simulink model "mcb_pmsm_param_est_f28379d"  (R2024b)
settings: Solver=FixedStepDiscrete  StartTime=0.0  StopTime=12  RelTol=1e-3  EnableMultiTasking=on
InitFcn:
  | mcb_pmsm_param_est_f28379d_data;
values from neighbouring files (symbols this model uses):
  dataType = 'single'    [mcb_pmsm_param_est_f28379d_data.m]
  inverter = evalin('base','inverter')    [mcb_param_est_StopFunc.m]    (also in mcb_pmsm_param_est_f28379d_data.m = mcb_updateInverterParameters(motor,inverter,target))
  target = mcb_SetProcessorDetails('F28379D',PWM_frequency)    [mcb_pmsm_param_est_f28379d_data.m]
  Ts = T_pwm    (= 5e-05)    [mcb_pmsm_param_est_f28379d_data.m]
  Ts_motor = T_pwm/2    (= 2.5e-05)    [mcb_pmsm_param_est_f28379d_data.m]
undefined symbols (not defined in the file or in its folder): Down, GPTRIP1SEL, GPTRIP2SEL, motor, TZ1, TZ2, Up
libraries: simulink x14, c2802xlib x8, c280xlib x5, mcbpmsmparamestlib x5, c2837xDlib x4, mcbpositiondecoderlib x3, svdschedulerlib x2, autolibpmsminterior x2, mcbplantlib x1, mcbcontrolslib x1, svdutilitieslib x1
(part 3 of 3)

== system mcb_pmsm_param_est_f28379d/Serial Receive/Variant Subsystem/Codegen/Subsystem/Switch Case Action Subsystem3 ==
  In1 : Inport
  Action Port : ActionPort
  Out1 : Outport
  wires:
  In1/1 -> Out1/1

== system mcb_pmsm_param_est_f28379d/Serial Receive/Variant Subsystem/Codegen/Subsystem/Switch Case Action Subsystem4 ==
  In1 : Inport
  Action Port : ActionPort
  Out1 : Outport
  wires:
  In1/1 -> Out1/1

== system mcb_pmsm_param_est_f28379d/Serial Receive/Variant Subsystem/Codegen/Subsystem/Switch Case Action Subsystem5 ==
  In1 : Inport
  Action Port : ActionPort
  Out1 : Outport
  wires:
  In1/1 -> Out1/1

== system mcb_pmsm_param_est_f28379d/Serial Receive/Variant Subsystem/Codegen/Subsystem/Switch Case Action Subsystem6 ==
  In1 : Inport
  Action Port : ActionPort
  Out1 : Outport
  wires:
  In1/1 -> Out1/1

== system mcb_pmsm_param_est_f28379d/Serial Receive/Variant Subsystem/Codegen/Subsystem/Switch Case Action Subsystem7 ==
  In1 : Inport
  Action Port : ActionPort
  Out1 : Outport
  wires:
  In1/1 -> Out1/1

== system mcb_pmsm_param_est_f28379d/Serial Receive/Variant Subsystem/Codegen/Subsystem/Switch Case Action Subsystem8 ==
  In1 : Inport
  Action Port : ActionPort  ActionPortLabel=case [ 21 ]:
  Out1 : Outport
  wires:
  In1/1 -> Out1/1

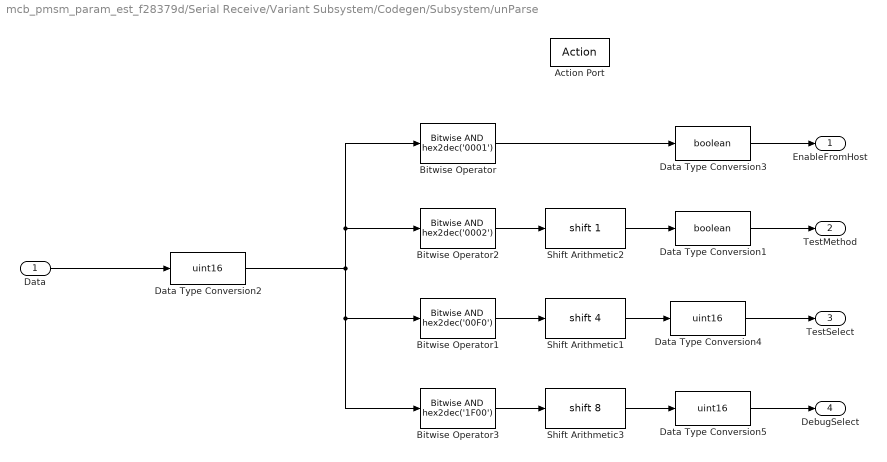
== system mcb_pmsm_param_est_f28379d/Serial Receive/Variant Subsystem/Codegen/Subsystem/unParse ==
  Data : Inport
  Action Port : ActionPort  ActionPortLabel=case [ 22 ]:
  Bitwise Operator : simulink/Logic and Bit Operations/Bitwise Operator  logicop=AND  UseBitMask=on  BitMask=hex2dec('0001')  BitMaskRealWorld=Stored Integer
  Bitwise Operator1 : simulink/Logic and Bit Operations/Bitwise Operator  logicop=AND  UseBitMask=on  BitMask=hex2dec('00F0')  BitMaskRealWorld=Stored Integer
  Bitwise Operator2 : simulink/Logic and Bit Operations/Bitwise Operator  logicop=AND  UseBitMask=on  BitMask=hex2dec('0002')  BitMaskRealWorld=Stored Integer
  Bitwise Operator3 : simulink/Logic and Bit Operations/Bitwise Operator  logicop=AND  UseBitMask=on  BitMask=hex2dec('1F00')  BitMaskRealWorld=Stored Integer
  Data Type Conversion1 : DataTypeConversion  OutDataTypeStr=boolean  RndMeth=Simplest  SaturateOnIntegerOverflow=off
  Data Type Conversion2 : DataTypeConversion  OutDataTypeStr=uint16  RndMeth=Simplest  SaturateOnIntegerOverflow=off
  Data Type Conversion3 : DataTypeConversion  OutDataTypeStr=boolean  RndMeth=Simplest  SaturateOnIntegerOverflow=off
  Data Type Conversion4 : DataTypeConversion  OutDataTypeStr=uint16  RndMeth=Simplest  SaturateOnIntegerOverflow=off
  Data Type Conversion5 : DataTypeConversion  OutDataTypeStr=uint16  RndMeth=Simplest  SaturateOnIntegerOverflow=off
  Shift Arithmetic1 : ArithShift  BitShiftNumber=4
  Shift Arithmetic2 : ArithShift  BitShiftNumber=1
  Shift Arithmetic3 : ArithShift  BitShiftNumber=8
  EnableFromHost : Outport
  TestMethod : Outport  Port=2
  TestSelect : Outport  Port=3
  DebugSelect : Outport  Port=4
  wires:
  Shift Arithmetic3/1 -> Data Type Conversion5/1
  Data Type Conversion5/1 -> DebugSelect/1
  Bitwise Operator3/1 -> Shift Arithmetic3/1
  Data Type Conversion2/1 -> Bitwise Operator1/1, Bitwise Operator3/1, Bitwise Operator/1, Bitwise Operator2/1
  Bitwise Operator1/1 -> Shift Arithmetic1/1
  Data/1 -> Data Type Conversion2/1
  Bitwise Operator/1 -> Data Type Conversion3/1
  Data Type Conversion4/1 -> TestSelect/1
  Shift Arithmetic1/1 -> Data Type Conversion4/1
  Data Type Conversion3/1 -> EnableFromHost/1
  Bitwise Operator2/1 -> Shift Arithmetic2/1
  Shift Arithmetic2/1 -> Data Type Conversion1/1
  Data Type Conversion1/1 -> TestMethod/1

== system mcb_pmsm_param_est_f28379d/Hardware Init/Variant Subsystem/Code Generation/Calculate ADC Offset /For Iterator Subsystem/If Action Subsystem ==
  In1 : Inport
  In2 : Inport  Port=2
  Action Port : ActionPort
  Memory : Memory  InheritSampleTime=on
  Memory1 : Memory  InheritSampleTime=on
  Sum : Sum
  Sum1 : Sum
  Out1 : Outport
  Out2 : Outport  Port=2
  wires:
  In1/1 -> Sum/1
  Sum/1 -> Out1/1, Memory/1
  In2/1 -> Sum1/1
  Memory/1 -> Sum/2
  Sum1/1 -> Out2/1, Memory1/1
  Memory1/1 -> Sum1/2

== system mcb_pmsm_param_est_f28379d/Parameter Estimation/Output HW Drivers/SCI Drivers/Codegen/Data_Conditioning_Tx/Data_Type_Fixed_Point ==
  In1 : Inport
  Data Type Conversion : DataTypeConversion  OutDataTypeStr=fixdt(1,32,28)  RndMeth=Simplest  SaturateOnIntegerOverflow=off
  Data Type Conversion3 : DataTypeConversion  OutDataTypeStr=uint32  ConvertRealWorld=Stored Integer (SI)  RndMeth=Simplest  SaturateOnIntegerOverflow=off
  Data_Log : Outport
  wires:
  In1/1 -> Data Type Conversion/1
  Data Type Conversion3/1 -> Data_Log/1
  Data Type Conversion/1 -> Data Type Conversion3/1

== system mcb_pmsm_param_est_f28379d/Parameter Estimation/Output HW Drivers/SCI Drivers/Codegen/Data_Conditioning_Tx/Data_Type_Float ==
  In1 : Inport
  Byte Pack : svdutilitieslib/Byte Pack  maskPackedDataType=uint32  datatypes={'single'}  byteAlign=4  blockPlatform=tic2000
  Data_Log : Outport
  wires:
  Byte Pack/1 -> Data_Log/1
  In1/1 -> Byte Pack/1

== system mcb_pmsm_param_est_f28379d/Parameter Estimation/Output HW Drivers/SCI Drivers/Codegen/Data_Logging/Data ==
  Data : Inport
  Data_width : Inport  Port=2
  Action Port : ActionPort  ActionPortLabel=else
  Dummy : Constant  Value=hex2dec('0000')  OutDataTypeStr=uint32
  Mux : Mux  Inputs=2
  Data_out : Outport  VectorParamsAs1DForOutWhenUnconnected=off
  Iteration : Outport  Port=2  VectorParamsAs1DForOutWhenUnconnected=off
  wires:
  Data_width/1 -> Iteration/1
  Data/1 -> Mux/1
  Dummy/1 -> Mux/2
  Mux/1 -> Data_out/1

== system mcb_pmsm_param_est_f28379d/Parameter Estimation/Output HW Drivers/SCI Drivers/Codegen/Data_Logging/End ==
  Data : Inport
  Data_width : Inport  Port=2
  Action Port : ActionPort  ActionPortLabel=elseif(u1 == 599)
  Bias : Bias  Bias=1  SaturateOnIntegerOverflow=off
  End : Constant  Value=hex2dec('45454545')  OutDataTypeStr=uint32
  Mux : Mux  Inputs=2
  Data_out : Outport  VectorParamsAs1DForOutWhenUnconnected=off
  Iteration : Outport  Port=2  VectorParamsAs1DForOutWhenUnconnected=off
  wires:
  Data/1 -> Mux/1
  Data_width/1 -> Bias/1
  Bias/1 -> Iteration/1
  End/1 -> Mux/2
  Mux/1 -> Data_out/1

== system mcb_pmsm_param_est_f28379d/Parameter Estimation/Output HW Drivers/SCI Drivers/Codegen/Data_Logging/Start ==
  Data : Inport
  Data_width : Inport  Port=2
  Action Port : ActionPort  ActionPortLabel=if(u1 == 0)
  Bias : Bias  Bias=1  SaturateOnIntegerOverflow=off
  Mux : Mux  Inputs=2
  Start : Constant  Value=hex2dec('53535353')  OutDataTypeStr=uint32
  Data_out : Outport  VectorParamsAs1DForOutWhenUnconnected=off
  Iteration : Outport  Port=2  VectorParamsAs1DForOutWhenUnconnected=off
  wires:
  Data/1 -> Mux/2
  Data_width/1 -> Bias/1
  Bias/1 -> Iteration/1
  Start/1 -> Mux/1
  Mux/1 -> Data_out/1

== stateflow chart mcb_pmsm_param_est_f28379d/Parameter Estimation/Param Est/Test Control/Chart ==
  state Init
    during: TestNum = uint16(0);
  state RsTestState
    during: TestNum = uint16(1);
  state LdTestState
    during: TestNum = uint16(2);
  state LqTestState1
    during: TestNum = uint16(3);
  state MechTestState
    during: TestNum = uint16(4);
  RsTestState -> Init [order 2] : [EnableIn == 0]
  (default) -> Init
  Init -> RsTestState : [EnableIn == 1 && EnPrev == 0]
  RsTestState -> LdTestState [order 1] : after(1/Ts,tick)[RsStatus == 2]
  MechTestState -> Init : after(1/Ts,tick)[MechStatus == 2]
  LqTestState1 -> Init [order 2] : [EnableIn == 0]
  LdTestState -> Init [order 2] : [EnableIn == 0]
  LdTestState -> LqTestState1 [order 1] : after(1/Ts,tick)[LdStatus == 2]
  LqTestState1 -> MechTestState [order 1] : after(1/Ts,tick)[LqStatus ==2]
  data: TestNum output; EnableIn input; EnPrev input; RsStatus input; LdStatus input; LqStatus input; MechStatus input; Ts input
